simulink model "bball"  (R2021a)
settings: Solver=ode15s  StartTime=0.0  StopTime=timeFinal  MaxStep=timeStepMax  RelTol=1e-3
undefined symbols (not defined in the file or in its folder): a1, a2
settings Model: Creator=amit  LastModifiedBy=amit

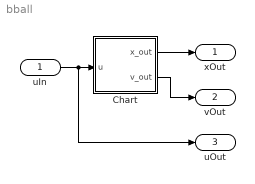
== system bball ==
  uIn : Inport
  Chart : Stateflow chart  TreatAsAtomicUnit=on
  xOut : Outport  SignalName=xOut
  vOut : Outport  Port=2  SignalName=vOut
  uOut : Outport  Port=3  SignalName=uOut
  wires:
  uIn/1 -> Chart/1(u), uOut/1
  Chart/2(v_out) -> vOut/1
  Chart/1(x_out) -> xOut/1

== stateflow chart bball/Chart ==
  settings: updateMethod=CONTINUOUS  executeAtInitialization=1
  state loc1
    du:
    x_dot = v;
    v_dot = -9.81 + 0.5 * u;
    exit:
    x_out = x;
    v_out = v;
  (default) -> loc1 : {x = a1; v = a2; }
  (junction 2) -> loc1 : [x <= 0 && v <= 0]{x = x; v = -0.75 * v; }
  loc1 -> (junction 2) [order 1]
  (junction 5) -> loc1 : [x >= 0.0]{x = x; v = v; }
  loc1 -> (junction 5) [order 2]
  data: u input; x_out output; v_out output; x local double; v local double; a1 parameter; a2 parameter
  data x settings: updateMethod=SF_CONTINUOUS_TIME_DATA
  data v settings: updateMethod=SF_CONTINUOUS_TIME_DATA
